simulink model "srm_simulink_template"  (R2020a)
settings: Solver=ode4  StartTime=0.0  StopTime=100  FixedStep=1E-3  RelTol=1e-3
libraries: robotmaniplib x1
settings Model: Creator=fernando  LastModifiedBy=fernando
settings SFSimCC: CustomCodeUndefinedFunction=UseInterfaceOnly

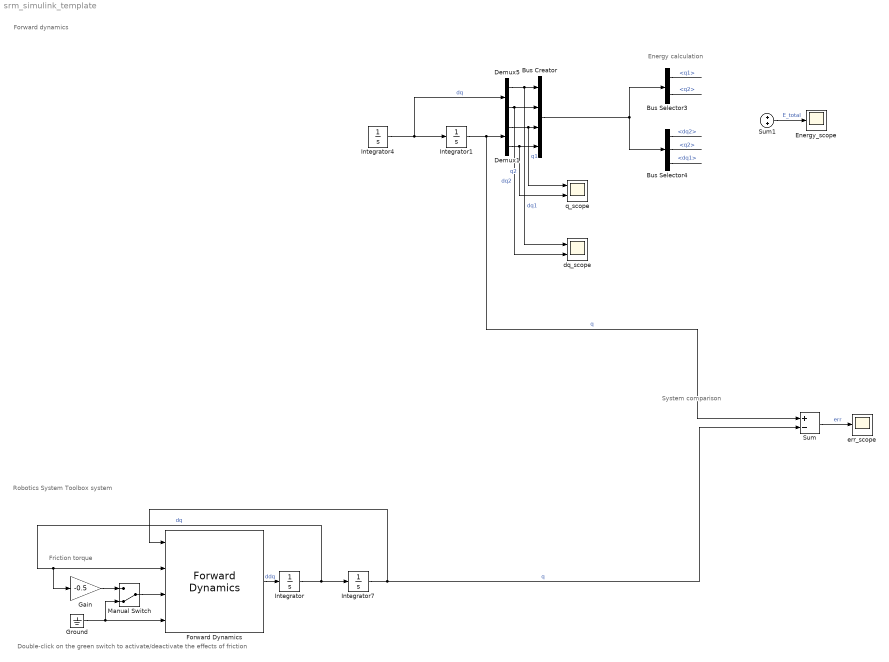
== system srm_simulink_template ==
  note: Double-click on the green switch to activate/deactivate the effects of friction
  note: Friction torque
  note: System comparison
  note: Robotics System Toolbox system
  note: Forward dynamics
  note: Energy calculation
  Bus Creator : BusCreator  Inputs=4
  Bus Selector3 : BusSelector  OutputSignals=q1,q2
  Bus Selector4 : BusSelector  OutputSignals=dq2,q2,dq1
  Demux1 : Demux  Outputs=2
  Demux5 : Demux  Outputs=2
  Energy_scope : Scope
  Forward Dynamics : robotmaniplib/Forward Dynamics  RigidBodyTree=twoLinkRobot  SimulateUsing=Code generation
  Gain : Gain  Gain=-0.5
  Ground : Ground
  Integrator : Integrator  InitialCondition=zeros(2,1)
  Integrator1 : Integrator  InitialCondition=[0 0]  WrapState=on
  Integrator4 : Integrator  InitialCondition=[0,0]
  Integrator7 : Integrator  InitialCondition=zeros(2,1)
  Manual Switch : ManualSwitch  CurrentSetting=0
  Sum : Sum  Inputs=+-
  Sum1 : Sum  Inputs=+|+
  dq_scope : Scope  NumInputPorts=2
  err_scope : Scope
  q_scope : Scope  NumInputPorts=2
  wires:
  Integrator4/1 -> Demux5/1, Integrator1/1  "dq"
  Integrator1/1 -> Sum/1, Demux1/1  "q"
  ? -> Integrator4/1  "ddq"
  ? -> Sum1/2  "T"
  Sum1/1 -> Energy_scope/1  "E_total"
  Demux5/1 -> dq_scope/1, Bus Creator/1  "dq1"
  Demux5/2 -> dq_scope/2, Bus Creator/2  "dq2"
  Demux1/1 -> q_scope/1, Bus Creator/3  "q1"
  Demux1/2 -> q_scope/2, Bus Creator/4  "q2"
  Bus Creator/1 -> Bus Selector3/1, Bus Selector4/1
  Bus Selector3/2 -> ?  "<q2>"
  Bus Selector3/1 -> ?  "<q1>"
  Bus Selector4/3 -> ?  "<dq1>"
  Bus Selector4/1 -> ?  "<dq2>"
  Bus Selector4/2 -> ?  "<q2>"
  ? -> Sum1/1  "U"
  Forward Dynamics/1 -> Integrator/1  "ddq"
  Integrator7/1 -> Forward Dynamics/1, Sum/2  "q"
  Ground/1 -> Forward Dynamics/4, Manual Switch/2
  Gain/1 -> Manual Switch/1
  Sum/1 -> err_scope/1  "err"
  Integrator/1 -> Forward Dynamics/2, Gain/1, Integrator7/1  "dq"
  Manual Switch/1 -> Forward Dynamics/3
